simulink model "ENV_NEW"  (R2024b)
settings: Solver=FixedStepDiscrete  StartTime=0.0  StopTime=1  FixedStep=0.001  RelTol=1e-3  EnableMultiTasking=on
libraries: stm32blockslib x105, canmsglib x32, stm32f4xxblockslib x11, simulink x10
(part 2 of 5)

== system ENV_NEW/CAN RX ==
  Digital Port Read5 : stm32f4xxblockslib/Digital Port Read  PortName=GPIOB  PinNumber=PinNumber  ReadOperation=on  IOAsArray=off  SampleTime=-1  EnableSimPort=off  hoistedMaskSrc=ECSoC/ECSimCodegen/Digital Port Read
      settings: LibrarySourceBlock=stm32f2xxblockslib/Digital Port Read
  Enabled Subsystem : Subsystem  TreatAsAtomicUnit=on
  NOT5 : Logic  Operator=NOT  IconShape=distinctive  AllPortsSameDT=off  OutDataTypeStr=boolean
  CANMessage : Outport
  wires:
  NOT5/1 -> Enabled Subsystem/Enable
  Digital Port Read5/1 -> NOT5/1
  Enabled Subsystem/1(CANMessage) -> CANMessage/1

== system ENV_NEW/CAN RX1 ==
  Digital Port Read5 : stm32f4xxblockslib/Digital Port Read  PortName=GPIOC  PinNumber=PinNumber  ReadOperation=on  IOAsArray=off  SampleTime=-1  EnableSimPort=off  hoistedMaskSrc=ECSoC/ECSimCodegen/Digital Port Read
      settings: LibrarySourceBlock=stm32f2xxblockslib/Digital Port Read
  Enabled Subsystem : Subsystem  TreatAsAtomicUnit=on
  NOT5 : Logic  Operator=NOT  IconShape=distinctive  AllPortsSameDT=off  OutDataTypeStr=boolean
  CANMessage : Outport
  wires:
  NOT5/1 -> Enabled Subsystem/Enable
  Digital Port Read5/1 -> NOT5/1
  Enabled Subsystem/1(CANMessage) -> CANMessage/1

== system ENV_NEW/CAN RX2 ==
  Digital Port Read5 : stm32f4xxblockslib/Digital Port Read  PortName=GPIOA  PinNumber=PinNumber  ReadOperation=on  IOAsArray=off  SampleTime=-1  EnableSimPort=off  hoistedMaskSrc=ECSoC/ECSimCodegen/Digital Port Read
      settings: LibrarySourceBlock=stm32f2xxblockslib/Digital Port Read
  Enabled Subsystem : Subsystem  TreatAsAtomicUnit=on
  NOT5 : Logic  Operator=NOT  IconShape=distinctive  AllPortsSameDT=off  OutDataTypeStr=boolean
  CANMessage : Outport
  wires:
  NOT5/1 -> Enabled Subsystem/Enable
  Digital Port Read5/1 -> NOT5/1
  Enabled Subsystem/1(CANMessage) -> CANMessage/1

== system ENV_NEW/CAN RX3 ==
  Digital Port Read5 : stm32f4xxblockslib/Digital Port Read  PortName=GPIOC  PinNumber=PinNumber  ReadOperation=on  IOAsArray=off  SampleTime=-1  EnableSimPort=off  hoistedMaskSrc=ECSoC/ECSimCodegen/Digital Port Read
      settings: LibrarySourceBlock=stm32f2xxblockslib/Digital Port Read
  Enabled Subsystem : Subsystem  TreatAsAtomicUnit=on
  NOT5 : Logic  Operator=NOT  IconShape=distinctive  AllPortsSameDT=off  OutDataTypeStr=boolean
  CANMessage : Outport
  wires:
  NOT5/1 -> Enabled Subsystem/Enable
  Digital Port Read5/1 -> NOT5/1
  Enabled Subsystem/1(CANMessage) -> CANMessage/1

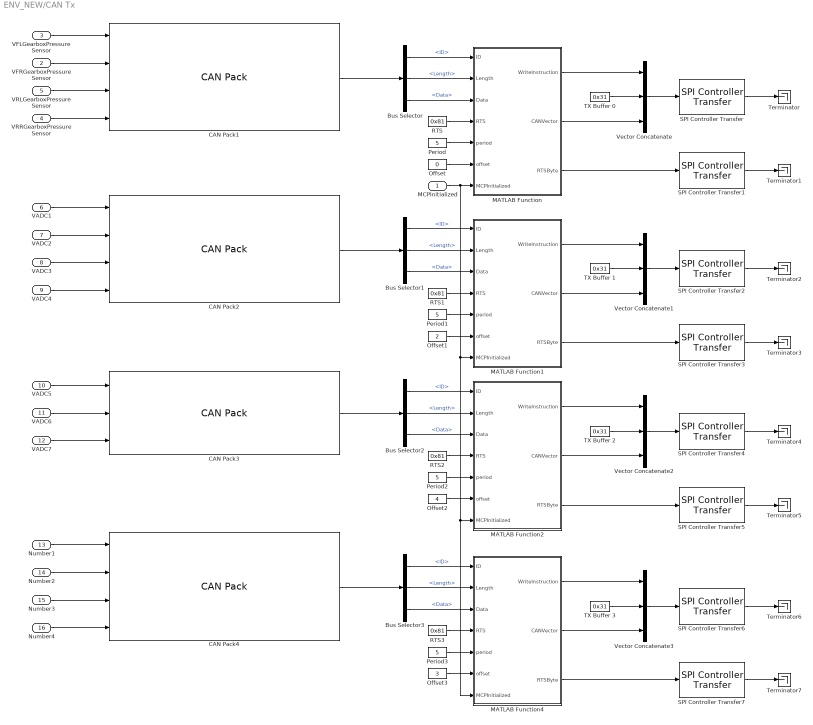
== system ENV_NEW/CAN Tx ==
  MCPInitialized : Inport
  VFRGearboxPressureSensor : Inport  Port=2
  VFLGearboxPressureSensor : Inport  Port=3
  VRRGearboxPressureSensor : Inport  Port=4
  VRLGearboxPressureSensor : Inport  Port=5
  VADC1 : Inport  Port=6
  VADC2 : Inport  Port=7
  VADC3 : Inport  Port=8
  VADC4 : Inport  Port=9
  VADC5 : Inport  Port=10
  VADC6 : Inport  Port=11
  VADC7 : Inport  Port=12
  Number1 : Inport  Port=13
  Number2 : Inport  Port=14
  Number3 : Inport  Port=15
  Number4 : Inport  Port=16
  Bus Selector{,1..3} (4 alike) : BusSelector  OutputSignals=ID,Length,Data
  CAN Pack1 : canmsglib/CAN Pack  CANdbFile=C:\Users\oxbro\Documents\STM32CustomProjects\PDUSTM32\ADCTest.dbc  MsgList=GearboxPressures  MsgName=GearboxPressures  MsgIDType=Standard (11-bit identifier)  MsgIdentifier=105  CANIDInput=off  MsgLength=8  Remote=off  ApplyMinMax=off  BusOutput=on  SignalInfo={'VFLGearboxPressureSensor','0','12','LE','unsigned','Standard','0','0.0012211','0','0','5.0004';'VFRGearboxPressureSensor','16','12','LE','unsigned','Standard','0','0.0012211','0','0','5.0004';'VRLGearboxPressureSensor','32','12','LE','unsigned','Standard','0','0.0012211','0','0','5.0004';'VRRGearboxPressureSensor','48','12','LE','unsigned','Standard','0','0.0012211','0','0','5.0004'}
      settings: LibrarySourceBlock=stmutilitieslib/CAN Pack  DataFormat=CANdb specified signals
  CAN Pack2 : canmsglib/CAN Pack  CANdbFile=C:\Users\oxbro\Documents\STM32CustomProjects\PDUSTM32\ADCTest.dbc  MsgList=ADCs1  MsgName=ADCs1  MsgIDType=Standard (11-bit identifier)  MsgIdentifier=5  CANIDInput=off  MsgLength=8  Remote=off  ApplyMinMax=off  BusOutput=on  SignalInfo={'VADC1','0','16','LE','unsigned','Standard','0','5.04e-05','0','0','3.303';'VADC2','16','16','LE','unsigned','Standard','0','5.04e-05','0','0','3.303';'VADC3','32','16','LE','unsigned','Standard','0','5.04e-05','0','0','3.303';'VADC4','48','16','LE','unsigned','Standard','0','5.04e-05','0','0','3.303'}
      settings: LibrarySourceBlock=stmutilitieslib/CAN Pack  DataFormat=CANdb specified signals
  CAN Pack3 : canmsglib/CAN Pack  CANdbFile=C:\Users\oxbro\Documents\STM32CustomProjects\PDUSTM32\ADCTest.dbc  MsgList=ADCs2  MsgName=ADCs2  MsgIDType=Standard (11-bit identifier)  MsgIdentifier=66  CANIDInput=off  MsgLength=6  Remote=off  ApplyMinMax=off  BusOutput=on  SignalInfo={'VADC5','0','16','LE','unsigned','Standard','0','5.04e-05','0','0','3.303';'VADC6','16','16','LE','unsigned','Standard','0','5.04e-05','0','0','3.303';'VLVSystem','32','16','LE','unsigned','Standard','0','0.00046327','0','0','30.3604'}
      settings: LibrarySourceBlock=stmutilitieslib/CAN Pack  DataFormat=CANdb specified signals
  CAN Pack4 : canmsglib/CAN Pack  CANdbFile=C:\Users\oxbro\Documents\STM32CustomProjects\PDUSTM32\ADCTest.dbc  MsgList=Numbers  MsgName=Numbers  MsgIDType=Standard (11-bit identifier)  MsgIdentifier=0  CANIDInput=off  MsgLength=8  Remote=off  ApplyMinMax=off  BusOutput=on  SignalInfo={'Number1','0','16','LE','signed','Standard','0','1','0','-32768','32767';'Number2','16','16','LE','signed','Standard','0','1','0','-32768','32767';'Number3','32','16','LE','signed','Standard','0','1','0','-32768','32767';'Number4','48','16','LE','signed','Standard','0','1','0','-32768','32767'}
      settings: LibrarySourceBlock=stmutilitieslib/CAN Pack  DataFormat=CANdb specified signals
  MATLAB Function : MATLAB Function  TreatAsAtomicUnit=on
  MATLAB Function1 : MATLAB Function  TreatAsAtomicUnit=on
  MATLAB Function2 : MATLAB Function  TreatAsAtomicUnit=on
  MATLAB Function4 : MATLAB Function  TreatAsAtomicUnit=on
  Offset : Constant  Value=0  OutDataTypeStr=uint16  SampleTime=-1
  Offset1 : Constant  Value=2  OutDataTypeStr=uint16  SampleTime=-1
  Offset2 : Constant  Value=4  OutDataTypeStr=uint16  SampleTime=-1
  Offset3 : Constant  Value=3  OutDataTypeStr=uint16  SampleTime=-1
  Period{,1..3} (4 alike) : Constant  Value=5  OutDataTypeStr=uint16  SampleTime=-1
  RTS{,1..3} (4 alike) : Constant  Value=0x81  OutDataTypeStr=uint8  SampleTime=-1
  SPI Controller Transfer{,2,4,6} (4 alike) : stm32blockslib/SPI Controller Transfer  Priority=1  SPIModuleSelect=SPI1  ClockPolarity=Low  ClockPhase=1 Edge  SPIModule=uint32(0)  Mode=Master  BusSpeed=uint32(1000000)  FirstBitToTransfer=Most significant bit (MSB)  ClockMode=0  BlockFunction=Transfer  EnableRegisterAddress=off  RegisterAddress=0  OutputDataType=uint8  OutputDataLength=1  OutputStatus=off  BlockingMode=off  Timeout=0.01  DataBits=8  UseCustomSSPin=Explicit GPIO calls  ActiveLowSSPin=Active low  Port_Select=GPIOA  Pin=1
      settings: LibrarySourceBlock=stm32h7xxblockslib/SPI Controller Transfer
  SPI Controller Transfer{1,3,5,7} (4 alike) : stm32blockslib/SPI Controller Transfer  Priority=2  SPIModuleSelect=SPI1  ClockPolarity=Low  ClockPhase=1 Edge  SPIModule=uint32(0)  Mode=Master  BusSpeed=uint32(1000000)  FirstBitToTransfer=Most significant bit (MSB)  ClockMode=0  BlockFunction=Transfer  EnableRegisterAddress=off  RegisterAddress=0  OutputDataType=uint8  OutputDataLength=1  OutputStatus=off  BlockingMode=off  Timeout=0.01  DataBits=8  UseCustomSSPin=Explicit GPIO calls  ActiveLowSSPin=Active low  Port_Select=GPIOA  Pin=1
      settings: LibrarySourceBlock=stm32h7xxblockslib/SPI Controller Transfer
  TX Buffer {0..3} (4 alike) : Constant  Value=0x31  OutDataTypeStr=uint8  SampleTime=-1
  Terminator{,1..7} (8 alike) : Terminator
  Vector Concatenate{,1..3} (4 alike) : Concatenate  NumInputs=3
  wires:
  SPI Controller Transfer/1 -> Terminator/1
  MATLAB Function/1(WriteInstruction) -> Vector Concatenate/1
  RTS/1 -> MATLAB Function/4(RTS)
  MATLAB Function/2(CANVector) -> Vector Concatenate/3
  SPI Controller Transfer1/1 -> Terminator1/1
  Bus Selector/1 -> MATLAB Function/1(ID)  "<ID>"
  Vector Concatenate/1 -> SPI Controller Transfer/1
  TX Buffer 0/1 -> Vector Concatenate/2
  MATLAB Function/3(RTSByte) -> SPI Controller Transfer1/1
  Bus Selector/2 -> MATLAB Function/2(Length)  "<Length>"
  Bus Selector/3 -> MATLAB Function/3(Data)  "<Data>"
  CAN Pack1/1 -> Bus Selector/1
  Period/1 -> MATLAB Function/5(period)
  Offset/1 -> MATLAB Function/6(offset)
  VRLGearboxPressureSensor/1 -> CAN Pack1/3
  VRRGearboxPressureSensor/1 -> CAN Pack1/4
  VFRGearboxPressureSensor/1 -> CAN Pack1/2
  VFLGearboxPressureSensor/1 -> CAN Pack1/1
  SPI Controller Transfer2/1 -> Terminator2/1
  SPI Controller Transfer3/1 -> Terminator3/1
  RTS1/1 -> MATLAB Function1/4(RTS)
  MATLAB Function1/2(CANVector) -> Vector Concatenate1/3
  Bus Selector1/3 -> MATLAB Function1/3(Data)  "<Data>"
  Period1/1 -> MATLAB Function1/5(period)
  Bus Selector1/2 -> MATLAB Function1/2(Length)  "<Length>"
  Offset1/1 -> MATLAB Function1/6(offset)
  CAN Pack2/1 -> Bus Selector1/1
  Bus Selector1/1 -> MATLAB Function1/1(ID)  "<ID>"
  MATLAB Function1/3(RTSByte) -> SPI Controller Transfer3/1
  Vector Concatenate1/1 -> SPI Controller Transfer2/1
  MATLAB Function1/1(WriteInstruction) -> Vector Concatenate1/1
  TX Buffer 1/1 -> Vector Concatenate1/2
  SPI Controller Transfer4/1 -> Terminator4/1
  SPI Controller Transfer5/1 -> Terminator5/1
  RTS2/1 -> MATLAB Function2/4(RTS)
  MATLAB Function2/2(CANVector) -> Vector Concatenate2/3
  Bus Selector2/3 -> MATLAB Function2/3(Data)  "<Data>"
  Period2/1 -> MATLAB Function2/5(period)
  Bus Selector2/2 -> MATLAB Function2/2(Length)  "<Length>"
  Offset2/1 -> MATLAB Function2/6(offset)
  CAN Pack3/1 -> Bus Selector2/1
  Bus Selector2/1 -> MATLAB Function2/1(ID)  "<ID>"
  MATLAB Function2/3(RTSByte) -> SPI Controller Transfer5/1
  Vector Concatenate2/1 -> SPI Controller Transfer4/1
  MATLAB Function2/1(WriteInstruction) -> Vector Concatenate2/1
  TX Buffer 2/1 -> Vector Concatenate2/2
  VADC1/1 -> CAN Pack2/1
  VADC2/1 -> CAN Pack2/2
  VADC3/1 -> CAN Pack2/3
  VADC4/1 -> CAN Pack2/4
  VADC5/1 -> CAN Pack3/1
  VADC6/1 -> CAN Pack3/2
  VADC7/1 -> CAN Pack3/3
  Period3/1 -> MATLAB Function4/5(period)
  Vector Concatenate3/1 -> SPI Controller Transfer6/1
  Offset3/1 -> MATLAB Function4/6(offset)
  Number1/1 -> CAN Pack4/1
  MATLAB Function4/3(RTSByte) -> SPI Controller Transfer7/1
  Number4/1 -> CAN Pack4/4
  MCPInitialized/1 -> MATLAB Function4/7(MCPInitialized), MATLAB Function2/7(MCPInitialized), MATLAB Function1/7(MCPInitialized), MATLAB Function/7(MCPInitialized)
  MATLAB Function4/2(CANVector) -> Vector Concatenate3/3
  Number3/1 -> CAN Pack4/3
  Bus Selector3/3 -> MATLAB Function4/3(Data)  "<Data>"
  Number2/1 -> CAN Pack4/2
  CAN Pack4/1 -> Bus Selector3/1
  Bus Selector3/1 -> MATLAB Function4/1(ID)  "<ID>"
  MATLAB Function4/1(WriteInstruction) -> Vector Concatenate3/1
  TX Buffer 3/1 -> Vector Concatenate3/2
  SPI Controller Transfer6/1 -> Terminator6/1
  SPI Controller Transfer7/1 -> Terminator7/1
  Bus Selector3/2 -> MATLAB Function4/2(Length)  "<Length>"
  RTS3/1 -> MATLAB Function4/4(RTS)

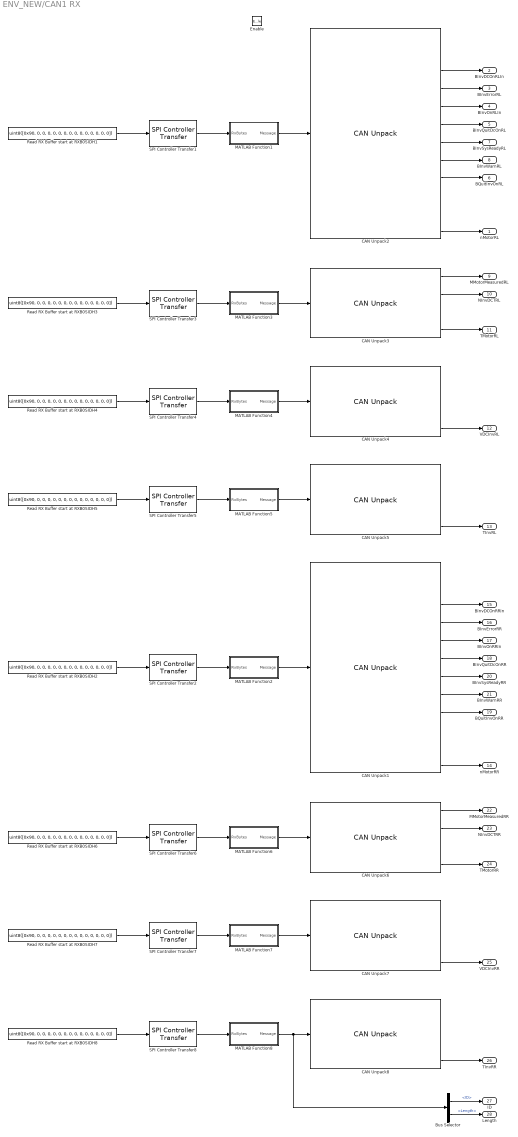
== system ENV_NEW/CAN1 RX ==
  Enable : EnablePort
  Bus Selector : BusSelector  OutputSignals=ID,Length
  CAN Unpack1 : canmsglib/CAN Unpack  CANdbFile=C:\Users\Will\Desktop\OBR\Embedded\VCUSTM32\Controls\CAN\Inverters\26.06.18_CAN1.dbc  MsgList=INV3_Send_1  MsgName=INV3_Send_1  MsgIDType=Standard (11-bit identifier)  MsgIdentifier=644  MsgLength=8  SignalInfo={'AMK_bDerating','47','1','LE','unsigned','Standard','0','1','0','0','1';'AMK_bReserve','32','8','LE','signed','Standard','0','1','0','-128','127';'BInvDCOnRRIn','44','1','LE','unsigned','Standard','0','1','0','0','1';'BInvErrorRR','41','1','LE','unsigned','Standard','0','1','0','0','1';'BInvOnRRIn','46','1','LE','unsigned','Standard','0','1','0','0','1';'BInvQuitDcOnRR','43','1','LE','unsigned','Standard','0','1','0','0','1';'BInvSysReadyRR','40','1','LE','unsigned','Standard','0','1','0','0','1';'BInvWarnRR','42','1','LE','unsigned','Standard','0','1','0','0','1';'BQuitInvOnRR','45','1','LE','unsigned','Standard','0','1','0','0','1';'Checksum','16','16','LE','unsigned','Standard','0','1','0','0','65535';'Message_Counter','0','16','LE','unsigned','Standard','0','1','0','0','65535';'nMotorRR','48','16','LE','signed','Standard','0','1','0','-32768','32767'}  IDPort=off  TimestampPort=off  ErrorPort=off  RemotePort=off  LengthPort=off  StatusPort=off  ApplyMinMax=off
      settings: LibrarySourceBlock=stmutilitieslib/CAN Unpack  DataFormat=CANdb specified signals
  CAN Unpack2 : canmsglib/CAN Unpack  CANdbFile=C:\Users\Will\Desktop\OBR\Embedded\VCUSTM32\Controls\CAN\Inverters\26.06.18_CAN1.dbc  MsgList=INV1_Send_1  MsgName=INV1_Send_1  MsgIDType=Standard (11-bit identifier)  MsgIdentifier=643  MsgLength=8  SignalInfo={'AMK_bDerating','47','1','LE','unsigned','Standard','0','1','0','0','1';'AMK_bReserve','32','8','LE','signed','Standard','0','1','0','-128','127';'BInvDCOnRLIn','44','1','LE','unsigned','Standard','0','1','0','0','1';'BInvErrorRL','41','1','LE','unsigned','Standard','0','1','0','0','1';'BInvOnRLIn','46','1','LE','unsigned','Standard','0','1','0','0','1';'BInvQuitDcOnRL','43','1','LE','unsigned','Standard','0','1','0','0','1';'BInvSysReadyRL','40','1','LE','unsigned','Standard','0','1','0','0','1';'BInvWarnRL','42','1','LE','unsigned','Standard','0','1','0','0','1';'BQuitInvOnRL','45','1','LE','unsigned','Standard','0','1','0','0','1';'Checksum','16','16','LE','unsigned','Standard','0','1','0','0','65535';'Message_Counter','0','16','LE','unsigned','Standard','0','1','0','0','65535';'nMotorRL','48','16','LE','signed','Standard','0','1','0','-32768','32767'}  IDPort=off  TimestampPort=off  ErrorPort=off  RemotePort=off  LengthPort=off  StatusPort=off  ApplyMinMax=off
      settings: LibrarySourceBlock=stmutilitieslib/CAN Unpack  DataFormat=CANdb specified signals
  CAN Unpack3 : canmsglib/CAN Unpack  CANdbFile=C:\Users\Will\Desktop\OBR\Embedded\VCUSTM32\Controls\CAN\Inverters\26.06.18_CAN1.dbc  MsgList=INV1_Send_2  MsgName=INV1_Send_2  MsgIDType=Standard (11-bit identifier)  MsgIdentifier=645  MsgLength=8  SignalInfo={'MMotorMeasuredRL','16','16','LE','signed','Standard','0','1','0','-32768','32767';'NInvDTCRL','32','16','LE','signed','Standard','0','1','0','-32768','32767';'NInvErrorInfoRL1','48','16','LE','signed','Standard','0','1','0','-32768','32767';'TMotorRL','0','16','LE','signed','Standard','0','0.1','0','-3276.8','3276.7'}  IDPort=off  TimestampPort=off  ErrorPort=off  RemotePort=off  LengthPort=off  StatusPort=off  ApplyMinMax=off
      settings: LibrarySourceBlock=stmutilitieslib/CAN Unpack  DataFormat=CANdb specified signals
  CAN Unpack4 : canmsglib/CAN Unpack  CANdbFile=C:\Users\Will\Desktop\OBR\Embedded\VCUSTM32\Controls\CAN\Inverters\26.06.18_CAN1.dbc  MsgList=INV1_Send_3  MsgName=INV1_Send_3  MsgIDType=Standard (11-bit identifier)  MsgIdentifier=647  MsgLength=8  SignalInfo={'NInvErrorInfoRL2','0','16','LE','signed','Standard','0','1','0','-32768','32767';'NInvErrorInfoRL3','16','16','LE','signed','Standard','0','1','0','-32768','32767';'Raw_Torque_Current','32','16','LE','signed','Standard','0','1','0','-32768','32767';'VDCInvRL','48','16','LE','signed','Standard','0','1','0','-32768','32767'}  IDPort=off  TimestampPort=off  ErrorPort=off  RemotePort=off  LengthPort=off  StatusPort=off  ApplyMinMax=off
      settings: LibrarySourceBlock=stmutilitieslib/CAN Unpack  DataFormat=CANdb specified signals
  CAN Unpack5 : canmsglib/CAN Unpack  CANdbFile=C:\Users\Will\Desktop\OBR\Embedded\VCUSTM32\Controls\CAN\Inverters\26.06.18_CAN1.dbc  MsgList=INV1_Send_4  MsgName=INV1_Send_4  MsgIDType=Standard (11-bit identifier)  MsgIdentifier=649  MsgLength=8  SignalInfo={'Converter_Peak_Current','32','16','LE','signed','Standard','0','1','0','-32768','32767';'Motor_Nomial_Current_IN','48','16','LE','signed','Standard','0','1','0','-32768','32767';'Motor_Peak_Current','16','16','LE','signed','Standard','0','1','0','-32768','32767';'TInvRL','0','16','LE','signed','Standard','0','0.1','0','-3276.8','3276.7'}  IDPort=off  TimestampPort=off  ErrorPort=off  RemotePort=off  LengthPort=off  StatusPort=off  ApplyMinMax=off
      settings: LibrarySourceBlock=stmutilitieslib/CAN Unpack  DataFormat=CANdb specified signals
  CAN Unpack6 : canmsglib/CAN Unpack  CANdbFile=C:\Users\Will\Desktop\OBR\Embedded\VCUSTM32\Controls\CAN\Inverters\26.06.18_CAN1.dbc  MsgList=INV3_Send_2  MsgName=INV3_Send_2  MsgIDType=Standard (11-bit identifier)  MsgIdentifier=646  MsgLength=8  SignalInfo={'MMotorMeasuredRR','16','16','LE','signed','Standard','0','1','0','-32768','32767';'NInvDTCRR','32','16','LE','signed','Standard','0','1','0','-32768','32767';'NInvErrorInfoRR1','48','16','LE','signed','Standard','0','1','0','-32768','32767';'TMotorRR','0','16','LE','signed','Standard','0','0.1','0','-3276.8','3276.7'}  IDPort=off  TimestampPort=off  ErrorPort=off  RemotePort=off  LengthPort=off  StatusPort=off  ApplyMinMax=off
      settings: LibrarySourceBlock=stmutilitieslib/CAN Unpack  DataFormat=CANdb specified signals
  CAN Unpack7 : canmsglib/CAN Unpack  CANdbFile=C:\Users\Will\Desktop\OBR\Embedded\VCUSTM32\Controls\CAN\Inverters\26.06.18_CAN1.dbc  MsgList=INV3_Send_3  MsgName=INV3_Send_3  MsgIDType=Standard (11-bit identifier)  MsgIdentifier=648  MsgLength=8  SignalInfo={'NInvErrorInfoRR2','0','16','LE','signed','Standard','0','1','0','-32768','32767';'NInvErrorInfoRR3','16','16','LE','signed','Standard','0','1','0','-32768','32767';'Raw_Torque_Current','32','16','LE','signed','Standard','0','1','0','-32768','32767';'VDCInvRR','48','16','LE','signed','Standard','0','1','0','-32768','32767'}  IDPort=off  TimestampPort=off  ErrorPort=off  RemotePort=off  LengthPort=off  StatusPort=off  ApplyMinMax=off
      settings: LibrarySourceBlock=stmutilitieslib/CAN Unpack  DataFormat=CANdb specified signals
  CAN Unpack8 : canmsglib/CAN Unpack  CANdbFile=C:\Users\Will\Desktop\OBR\Embedded\VCUSTM32\Controls\CAN\Inverters\26.06.18_CAN1.dbc  MsgList=INV3_Send_4  MsgName=INV3_Send_4  MsgIDType=Standard (11-bit identifier)  MsgIdentifier=656  MsgLength=8  SignalInfo={'Converter_Peak_Current','32','16','LE','signed','Standard','0','1','0','-32768','32767';'Motor_Nomial_Current_IN','48','16','LE','signed','Standard','0','1','0','-32768','32767';'Motor_Peak_Current','16','16','LE','signed','Standard','0','1','0','-32768','32767';'TInvRR','0','16','LE','signed','Standard','0','0.1','0','-3276.8','3276.7'}  IDPort=off  TimestampPort=off  ErrorPort=off  RemotePort=off  LengthPort=off  StatusPort=off  ApplyMinMax=off
      settings: LibrarySourceBlock=stmutilitieslib/CAN Unpack  DataFormat=CANdb specified signals
  MATLAB Function1 : MATLAB Function  TreatAsAtomicUnit=on
  MATLAB Function2 : MATLAB Function  TreatAsAtomicUnit=on
  MATLAB Function3 : MATLAB Function  TreatAsAtomicUnit=on
  MATLAB Function4 : MATLAB Function  TreatAsAtomicUnit=on
  MATLAB Function5 : MATLAB Function  TreatAsAtomicUnit=on
  MATLAB Function6 : MATLAB Function  TreatAsAtomicUnit=on
  MATLAB Function7 : MATLAB Function  TreatAsAtomicUnit=on
  MATLAB Function8 : MATLAB Function  TreatAsAtomicUnit=on
  Read RX Buffer start at RXB0SIDH{1..8} (8 alike) : Constant  Value=uint8([0x90, 0, 0, 0, 0, 0, 0, 0, 0, 0, 0, 0, 0, 0, 0])
  SPI Controller Transfer{1..8} (8 alike) : stm32blockslib/SPI Controller Transfer  Priority=1  SPIModuleSelect=SPI1  ClockPolarity=Low  ClockPhase=1 Edge  SPIModule=uint32(0)  Mode=Master  BusSpeed=uint32(1000000)  FirstBitToTransfer=Most significant bit (MSB)  ClockMode=0  BlockFunction=Transfer  EnableRegisterAddress=off  RegisterAddress=0  OutputDataType=uint8  OutputDataLength=1  OutputStatus=off  BlockingMode=on  Timeout=0.01  DataBits=8  UseCustomSSPin=Explicit GPIO calls  ActiveLowSSPin=Active low  Port_Select=GPIOB  Pin=1
      settings: LibrarySourceBlock=stm32h7xxblockslib/SPI Controller Transfer
  nMotorRL : Outport  OutDataTypeStr=double
  BInvDCOnRLIn : Outport  Port=2  OutDataTypeStr=boolean
  BInvErrorRL : Outport  Port=3  OutDataTypeStr=boolean
  BInvOnRLIn : Outport  Port=4  OutDataTypeStr=boolean
  BInvQuitDcOnRL : Outport  Port=5  OutDataTypeStr=boolean
  BQuitInvOnRL : Outport  Port=6  OutDataTypeStr=boolean
  BInvSysReadyRL : Outport  Port=7  OutDataTypeStr=boolean
  BInvWarnRL : Outport  Port=8  OutDataTypeStr=boolean
  MMotorMeasuredRL : Outport  Port=9  OutDataTypeStr=double
  NInvDCTRL : Outport  Port=10  OutDataTypeStr=double
  TMotorRL : Outport  Port=11  OutDataTypeStr=double
  VDCInvRL : Outport  Port=12  OutDataTypeStr=double
  TInvRL : Outport  Port=13  OutDataTypeStr=double
  nMotorRR : Outport  Port=14  OutDataTypeStr=double
  BInvDCOnRRIn : Outport  Port=15  OutDataTypeStr=boolean
  BInvErrorRR : Outport  Port=16  OutDataTypeStr=boolean
  BInvOnRRIn : Outport  Port=17  OutDataTypeStr=boolean
  BInvQuitDcOnRR : Outport  Port=18  OutDataTypeStr=boolean
  BQuitInvOnRR : Outport  Port=19  OutDataTypeStr=boolean
  BInvSysReadyRR : Outport  Port=20  OutDataTypeStr=boolean
  BInvWarnRR : Outport  Port=21  OutDataTypeStr=boolean
  MMotorMeasuredRR : Outport  Port=22  OutDataTypeStr=double
  NInvDCTRR : Outport  Port=23  OutDataTypeStr=double
  TMotorRR : Outport  Port=24  OutDataTypeStr=double
  VDCInvRR : Outport  Port=25  OutDataTypeStr=double
  TInvRR : Outport  Port=26  OutDataTypeStr=double
  ID : Outport  Port=27
  Length : Outport  Port=28
  wires:
  Read RX Buffer start at RXB0SIDH1/1 -> SPI Controller Transfer1/1
  SPI Controller Transfer1/1 -> MATLAB Function1/1(RxBytes)
  MATLAB Function1/1(Message) -> CAN Unpack2/1
  CAN Unpack2/3 -> BInvDCOnRLIn/1
  CAN Unpack2/4 -> BInvErrorRL/1
  CAN Unpack2/5 -> BInvOnRLIn/1
  CAN Unpack2/6 -> BInvQuitDcOnRL/1
  CAN Unpack2/9 -> BQuitInvOnRL/1
  CAN Unpack2/8 -> BInvWarnRL/1
  CAN Unpack2/7 -> BInvSysReadyRL/1
  CAN Unpack2/12 -> nMotorRL/1
  CAN Unpack3/4 -> TMotorRL/1
  MATLAB Function3/1(Message) -> CAN Unpack3/1
  SPI Controller Transfer3/1 -> MATLAB Function3/1(RxBytes)
  Read RX Buffer start at RXB0SIDH3/1 -> SPI Controller Transfer3/1
  CAN Unpack3/1 -> MMotorMeasuredRL/1
  CAN Unpack3/2 -> NInvDCTRL/1
  CAN Unpack4/4 -> VDCInvRL/1
  SPI Controller Transfer4/1 -> MATLAB Function4/1(RxBytes)
  MATLAB Function4/1(Message) -> CAN Unpack4/1
  Read RX Buffer start at RXB0SIDH4/1 -> SPI Controller Transfer4/1
  SPI Controller Transfer5/1 -> MATLAB Function5/1(RxBytes)
  CAN Unpack5/4 -> TInvRL/1
  Read RX Buffer start at RXB0SIDH5/1 -> SPI Controller Transfer5/1
  MATLAB Function5/1(Message) -> CAN Unpack5/1
  MATLAB Function8/1(Message) -> CAN Unpack8/1, Bus Selector/1
  Bus Selector/2 -> Length/1  "<Length>"
  Bus Selector/1 -> ID/1  "<ID>"
  CAN Unpack1/6 -> BInvQuitDcOnRR/1
  CAN Unpack1/3 -> BInvDCOnRRIn/1
  CAN Unpack6/4 -> TMotorRR/1
  CAN Unpack1/5 -> BInvOnRRIn/1
  SPI Controller Transfer2/1 -> MATLAB Function2/1(RxBytes)
  MATLAB Function2/1(Message) -> CAN Unpack1/1
  SPI Controller Transfer8/1 -> MATLAB Function8/1(RxBytes)
  CAN Unpack1/8 -> BInvWarnRR/1
  CAN Unpack6/1 -> MMotorMeasuredRR/1
  CAN Unpack1/12 -> nMotorRR/1
  CAN Unpack1/4 -> BInvErrorRR/1
  CAN Unpack1/7 -> BInvSysReadyRR/1
  CAN Unpack1/9 -> BQuitInvOnRR/1
  Read RX Buffer start at RXB0SIDH2/1 -> SPI Controller Transfer2/1
  SPI Controller Transfer7/1 -> MATLAB Function7/1(RxBytes)
  Read RX Buffer start at RXB0SIDH8/1 -> SPI Controller Transfer8/1
  MATLAB Function6/1(Message) -> CAN Unpack6/1
  Read RX Buffer start at RXB0SIDH7/1 -> SPI Controller Transfer7/1
  CAN Unpack6/2 -> NInvDCTRR/1
  SPI Controller Transfer6/1 -> MATLAB Function6/1(RxBytes)
  MATLAB Function7/1(Message) -> CAN Unpack7/1
  Read RX Buffer start at RXB0SIDH6/1 -> SPI Controller Transfer6/1
  CAN Unpack7/4 -> VDCInvRR/1
  CAN Unpack8/4 -> TInvRR/1

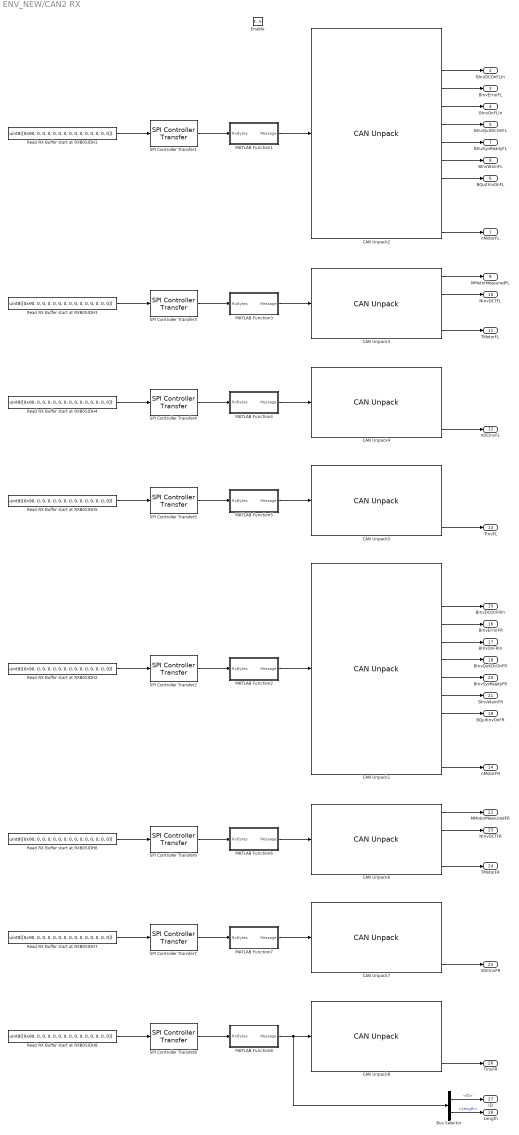
== system ENV_NEW/CAN2 RX ==
  Enable : EnablePort
  Bus Selector : BusSelector  OutputSignals=ID,Length
  CAN Unpack1 : canmsglib/CAN Unpack  CANdbFile=C:\Users\Will\Desktop\OBR\Embedded\VCUSTM32\Controls\CAN\Inverters\26.06.18_CAN2.dbc  MsgList=INV4_Send_1  MsgName=INV4_Send_1  MsgIDType=Standard (11-bit identifier)  MsgIdentifier=658  MsgLength=8  SignalInfo={'AMK_bDerating','47','1','LE','unsigned','Standard','0','1','0','0','1';'AMK_bReserve','32','8','LE','signed','Standard','0','1','0','-128','127';'BInvDCOnFRIn','44','1','LE','unsigned','Standard','0','1','0','0','1';'BInvErrorFR','41','1','LE','unsigned','Standard','0','1','0','0','1';'BInvOnFRIn','46','1','LE','unsigned','Standard','0','1','0','0','1';'BInvQuitDcOnFR','43','1','LE','unsigned','Standard','0','1','0','0','1';'BInvSysReadyFR','40','1','LE','unsigned','Standard','0','1','0','0','1';'BInvWarnFR','42','1','LE','unsigned','Standard','0','1','0','0','1';'BQuitInvOnFR','45','1','LE','unsigned','Standard','0','1','0','0','1';'Checksum','16','16','LE','unsigned','Standard','0','1','0','0','65535';'Message_Counter','0','16','LE','unsigned','Standard','0','1','0','0','65535';'nMotorFR','48','16','LE','signed','Standard','0','1','0','-32768','32767'}  IDPort=off  TimestampPort=off  ErrorPort=off  RemotePort=off  LengthPort=off  StatusPort=off  ApplyMinMax=off
      settings: LibrarySourceBlock=stmutilitieslib/CAN Unpack  DataFormat=CANdb specified signals
  CAN Unpack2 : canmsglib/CAN Unpack  CANdbFile=C:\Users\Will\Desktop\OBR\Embedded\VCUSTM32\Controls\CAN\Inverters\26.06.18_CAN2.dbc  MsgList=INV2_Send_1  MsgName=INV2_Send_1  MsgIDType=Standard (11-bit identifier)  MsgIdentifier=657  MsgLength=8  SignalInfo={'AMK_bDerating','47','1','LE','unsigned','Standard','0','1','0','0','1';'AMK_bReserve','32','8','LE','signed','Standard','0','1','0','-128','127';'BInvDCOnFLIn','44','1','LE','unsigned','Standard','0','1','0','0','1';'BInvErrorFL','41','1','LE','unsigned','Standard','0','1','0','0','1';'BInvOnFLIn','46','1','LE','unsigned','Standard','0','1','0','0','1';'BInvQuitDcOnFL','43','1','LE','unsigned','Standard','0','1','0','0','1';'BInvSysReadyFL','40','1','LE','unsigned','Standard','0','1','0','0','1';'BInvWarnFL','42','1','LE','unsigned','Standard','0','1','0','0','1';'BQuitInvOnFL','45','1','LE','unsigned','Standard','0','1','0','0','1';'Checksum','16','16','LE','unsigned','Standard','0','1','0','0','65535';'Message_Counter','0','16','LE','unsigned','Standard','0','1','0','0','65535';'nMotorFL','48','16','LE','signed','Standard','0','1','0','-32768','32767'}  IDPort=off  TimestampPort=off  ErrorPort=off  RemotePort=off  LengthPort=off  StatusPort=off  ApplyMinMax=off
      settings: LibrarySourceBlock=stmutilitieslib/CAN Unpack  DataFormat=CANdb specified signals
  CAN Unpack3 : canmsglib/CAN Unpack  CANdbFile=C:\Users\Will\Desktop\OBR\Embedded\VCUSTM32\Controls\CAN\Inverters\26.06.18_CAN2.dbc  MsgList=INV2_Send_2  MsgName=INV2_Send_2  MsgIDType=Standard (11-bit identifier)  MsgIdentifier=659  MsgLength=8  SignalInfo={'MMotorMeasuredFL','16','16','LE','signed','Standard','0','1','0','-32768','32767';'NInvDTCFL','32','16','LE','signed','Standard','0','1','0','-32768','32767';'NInvErrorInfoFL1','48','16','LE','signed','Standard','0','1','0','-32768','32767';'TMotorFL','0','16','LE','signed','Standard','0','0.1','0','-3276.8','3276.7'}  IDPort=off  TimestampPort=off  ErrorPort=off  RemotePort=off  LengthPort=off  StatusPort=off  ApplyMinMax=off
      settings: LibrarySourceBlock=stmutilitieslib/CAN Unpack  DataFormat=CANdb specified signals
  CAN Unpack4 : canmsglib/CAN Unpack  CANdbFile=C:\Users\Will\Desktop\OBR\Embedded\VCUSTM32\Controls\CAN\Inverters\26.06.18_CAN2.dbc  MsgList=INV2_Send_3  MsgName=INV2_Send_3  MsgIDType=Standard (11-bit identifier)  MsgIdentifier=661  MsgLength=8  SignalInfo={'NInvErrorInfoFL2','0','16','LE','signed','Standard','0','1','0','-32768','32767';'NInvErrorInfoFL3','16','16','LE','signed','Standard','0','1','0','-32768','32767';'Raw_Torque_Current','32','16','LE','signed','Standard','0','1','0','-32768','32767';'VDCInvFL','48','16','LE','signed','Standard','0','1','0','-32768','32767'}  IDPort=off  TimestampPort=off  ErrorPort=off  RemotePort=off  LengthPort=off  StatusPort=off  ApplyMinMax=off
      settings: LibrarySourceBlock=stmutilitieslib/CAN Unpack  DataFormat=CANdb specified signals
  CAN Unpack5 : canmsglib/CAN Unpack  CANdbFile=C:\Users\Will\Desktop\OBR\Embedded\VCUSTM32\Controls\CAN\Inverters\26.06.18_CAN2.dbc  MsgList=INV2_Send_4  MsgName=INV2_Send_4  MsgIDType=Standard (11-bit identifier)  MsgIdentifier=663  MsgLength=8  SignalInfo={'Converter_Peak_Current','32','16','LE','signed','Standard','0','1','0','-32768','32767';'Motor_Nomial_Current_IN','48','16','LE','signed','Standard','0','1','0','-32768','32767';'Motor_Peak_Current','16','16','LE','signed','Standard','0','1','0','-32768','32767';'TInvFL','0','16','LE','signed','Standard','0','0.1','0','-3276.8','3276.7'}  IDPort=off  TimestampPort=off  ErrorPort=off  RemotePort=off  LengthPort=off  StatusPort=off  ApplyMinMax=off
      settings: LibrarySourceBlock=stmutilitieslib/CAN Unpack  DataFormat=CANdb specified signals
  CAN Unpack6 : canmsglib/CAN Unpack  CANdbFile=C:\Users\Will\Desktop\OBR\Embedded\VCUSTM32\Controls\CAN\Inverters\26.06.18_CAN2.dbc  MsgList=INV4_Send_2  MsgName=INV4_Send_2  MsgIDType=Standard (11-bit identifier)  MsgIdentifier=660  MsgLength=8  SignalInfo={'MMotorMeasuredFR','16','16','LE','signed','Standard','0','1','0','-32768','32767';'NInvDTCFR','32','16','LE','signed','Standard','0','1','0','-32768','32767';'NInvErrorInfoFR1','48','16','LE','signed','Standard','0','1','0','-32768','32767';'TMotorFR','0','16','LE','signed','Standard','0','0.1','0','-3276.8','3276.7'}  IDPort=off  TimestampPort=off  ErrorPort=off  RemotePort=off  LengthPort=off  StatusPort=off  ApplyMinMax=off
      settings: LibrarySourceBlock=stmutilitieslib/CAN Unpack  DataFormat=CANdb specified signals
  CAN Unpack7 : canmsglib/CAN Unpack  CANdbFile=C:\Users\Will\Desktop\OBR\Embedded\VCUSTM32\Controls\CAN\Inverters\26.06.18_CAN2.dbc  MsgList=INV4_Send_3  MsgName=INV4_Send_3  MsgIDType=Standard (11-bit identifier)  MsgIdentifier=662  MsgLength=8  SignalInfo={'NInvErrorInfoFR2','0','16','LE','signed','Standard','0','1','0','-32768','32767';'NInvErrorInfoFR3','16','16','LE','signed','Standard','0','1','0','-32768','32767';'Raw_Torque_Current','32','16','LE','signed','Standard','0','1','0','-32768','32767';'VDCInvFR','48','16','LE','signed','Standard','0','1','0','-32768','32767'}  IDPort=off  TimestampPort=off  ErrorPort=off  RemotePort=off  LengthPort=off  StatusPort=off  ApplyMinMax=off
      settings: LibrarySourceBlock=stmutilitieslib/CAN Unpack  DataFormat=CANdb specified signals
  CAN Unpack8 : canmsglib/CAN Unpack  CANdbFile=C:\Users\Will\Desktop\OBR\Embedded\VCUSTM32\Controls\CAN\Inverters\26.06.18_CAN2.dbc  MsgList=INV4_Send_4  MsgName=INV4_Send_4  MsgIDType=Standard (11-bit identifier)  MsgIdentifier=664  MsgLength=8  SignalInfo={'Converter_Peak_Current','32','16','LE','signed','Standard','0','1','0','-32768','32767';'Motor_Nomial_Current_IN','48','16','LE','signed','Standard','0','1','0','-32768','32767';'Motor_Peak_Current','16','16','LE','signed','Standard','0','1','0','-32768','32767';'TInvFR','0','16','LE','signed','Standard','0','0.1','0','-3276.8','3276.7'}  IDPort=off  TimestampPort=off  ErrorPort=off  RemotePort=off  LengthPort=off  StatusPort=off  ApplyMinMax=off
      settings: LibrarySourceBlock=stmutilitieslib/CAN Unpack  DataFormat=CANdb specified signals
  MATLAB Function1 : MATLAB Function  TreatAsAtomicUnit=on
  MATLAB Function2 : MATLAB Function  TreatAsAtomicUnit=on
  MATLAB Function3 : MATLAB Function  TreatAsAtomicUnit=on
  MATLAB Function4 : MATLAB Function  TreatAsAtomicUnit=on
  MATLAB Function5 : MATLAB Function  TreatAsAtomicUnit=on
  MATLAB Function6 : MATLAB Function  TreatAsAtomicUnit=on
  MATLAB Function7 : MATLAB Function  TreatAsAtomicUnit=on
  MATLAB Function8 : MATLAB Function  TreatAsAtomicUnit=on
  Read RX Buffer start at RXB0SIDH{1..8} (8 alike) : Constant  Value=uint8([0x90, 0, 0, 0, 0, 0, 0, 0, 0, 0, 0, 0, 0, 0, 0])
  SPI Controller Transfer{1..8} (8 alike) : stm32blockslib/SPI Controller Transfer  Priority=1  SPIModuleSelect=SPI1  ClockPolarity=Low  ClockPhase=1 Edge  SPIModule=uint32(0)  Mode=Master  BusSpeed=uint32(1000000)  FirstBitToTransfer=Most significant bit (MSB)  ClockMode=0  BlockFunction=Transfer  EnableRegisterAddress=off  RegisterAddress=0  OutputDataType=uint8  OutputDataLength=1  OutputStatus=off  BlockingMode=on  Timeout=0.01  DataBits=8  UseCustomSSPin=Explicit GPIO calls  ActiveLowSSPin=Active low  Port_Select=GPIOC  Pin=10
      settings: LibrarySourceBlock=stm32h7xxblockslib/SPI Controller Transfer
  nMotorFL : Outport  OutDataTypeStr=double
  BInvDCOnFLIn : Outport  Port=2  OutDataTypeStr=boolean
  BInvErrorFL : Outport  Port=3  OutDataTypeStr=boolean
  BInvOnFLIn : Outport  Port=4  OutDataTypeStr=boolean
  BInvQuitDcOnFL : Outport  Port=5  OutDataTypeStr=boolean
  BQuitInvOnFL : Outport  Port=6  OutDataTypeStr=boolean
  BInvSysReadyFL : Outport  Port=7  OutDataTypeStr=boolean
  BInvWarnFL : Outport  Port=8  OutDataTypeStr=boolean
  MMotorMeasuredFL : Outport  Port=9  OutDataTypeStr=double
  NInvDCTFL : Outport  Port=10  OutDataTypeStr=double
  TMotorFL : Outport  Port=11  OutDataTypeStr=double
  VDCInvFL : Outport  Port=12  OutDataTypeStr=double
  TInvFL : Outport  Port=13  OutDataTypeStr=double
  nMotorFR : Outport  Port=14  OutDataTypeStr=double
  BInvDCOnFRIn : Outport  Port=15  OutDataTypeStr=boolean
  BInvErrorFR : Outport  Port=16  OutDataTypeStr=boolean
  BInvOnFRIn : Outport  Port=17  OutDataTypeStr=boolean
  BInvQuitDcOnFR : Outport  Port=18  OutDataTypeStr=boolean
  BQuitInvOnFR : Outport  Port=19  OutDataTypeStr=boolean
  BInvSysReadyFR : Outport  Port=20  OutDataTypeStr=boolean
  BInvWarnFR : Outport  Port=21  OutDataTypeStr=boolean
  MMotorMeasuredFR : Outport  Port=22  OutDataTypeStr=double
  NInvDCTFR : Outport  Port=23  OutDataTypeStr=double
  TMotorFR : Outport  Port=24  OutDataTypeStr=double
  VDCInvFR : Outport  Port=25  OutDataTypeStr=double
  TInvFR : Outport  Port=26  OutDataTypeStr=double
  ID : Outport  Port=27
  Length : Outport  Port=28
  wires:
  Read RX Buffer start at RXB0SIDH1/1 -> SPI Controller Transfer1/1
  SPI Controller Transfer1/1 -> MATLAB Function1/1(RxBytes)
  MATLAB Function1/1(Message) -> CAN Unpack2/1
  CAN Unpack2/3 -> BInvDCOnFLIn/1
  CAN Unpack2/4 -> BInvErrorFL/1
  CAN Unpack2/5 -> BInvOnFLIn/1
  CAN Unpack2/6 -> BInvQuitDcOnFL/1
  CAN Unpack2/9 -> BQuitInvOnFL/1
  CAN Unpack2/8 -> BInvWarnFL/1
  CAN Unpack2/7 -> BInvSysReadyFL/1
  CAN Unpack2/12 -> nMotorFL/1
  CAN Unpack3/4 -> TMotorFL/1
  MATLAB Function3/1(Message) -> CAN Unpack3/1
  SPI Controller Transfer3/1 -> MATLAB Function3/1(RxBytes)
  Read RX Buffer start at RXB0SIDH3/1 -> SPI Controller Transfer3/1
  CAN Unpack3/1 -> MMotorMeasuredFL/1
  CAN Unpack3/2 -> NInvDCTFL/1
  CAN Unpack4/4 -> VDCInvFL/1
  SPI Controller Transfer4/1 -> MATLAB Function4/1(RxBytes)
  MATLAB Function4/1(Message) -> CAN Unpack4/1
  Read RX Buffer start at RXB0SIDH4/1 -> SPI Controller Transfer4/1
  SPI Controller Transfer5/1 -> MATLAB Function5/1(RxBytes)
  CAN Unpack5/4 -> TInvFL/1
  Read RX Buffer start at RXB0SIDH5/1 -> SPI Controller Transfer5/1
  MATLAB Function5/1(Message) -> CAN Unpack5/1
  MATLAB Function8/1(Message) -> Bus Selector/1, CAN Unpack8/1
  Bus Selector/2 -> Length/1  "<Length>"
  Bus Selector/1 -> ID/1  "<ID>"
  CAN Unpack1/6 -> BInvQuitDcOnFR/1
  CAN Unpack1/3 -> BInvDCOnFRIn/1
  CAN Unpack6/4 -> TMotorFR/1
  CAN Unpack1/5 -> BInvOnFRIn/1
  SPI Controller Transfer2/1 -> MATLAB Function2/1(RxBytes)
  MATLAB Function2/1(Message) -> CAN Unpack1/1
  SPI Controller Transfer8/1 -> MATLAB Function8/1(RxBytes)
  CAN Unpack1/8 -> BInvWarnFR/1
  CAN Unpack6/1 -> MMotorMeasuredFR/1
  CAN Unpack1/12 -> nMotorFR/1
  CAN Unpack1/4 -> BInvErrorFR/1
  CAN Unpack1/7 -> BInvSysReadyFR/1
  CAN Unpack1/9 -> BQuitInvOnFR/1
  Read RX Buffer start at RXB0SIDH2/1 -> SPI Controller Transfer2/1
  SPI Controller Transfer7/1 -> MATLAB Function7/1(RxBytes)
  Read RX Buffer start at RXB0SIDH8/1 -> SPI Controller Transfer8/1
  MATLAB Function6/1(Message) -> CAN Unpack6/1
  Read RX Buffer start at RXB0SIDH7/1 -> SPI Controller Transfer7/1
  CAN Unpack6/2 -> NInvDCTFR/1
  SPI Controller Transfer6/1 -> MATLAB Function6/1(RxBytes)
  MATLAB Function7/1(Message) -> CAN Unpack7/1
  Read RX Buffer start at RXB0SIDH6/1 -> SPI Controller Transfer6/1
  CAN Unpack7/4 -> VDCInvFR/1
  CAN Unpack8/4 -> TInvFR/1

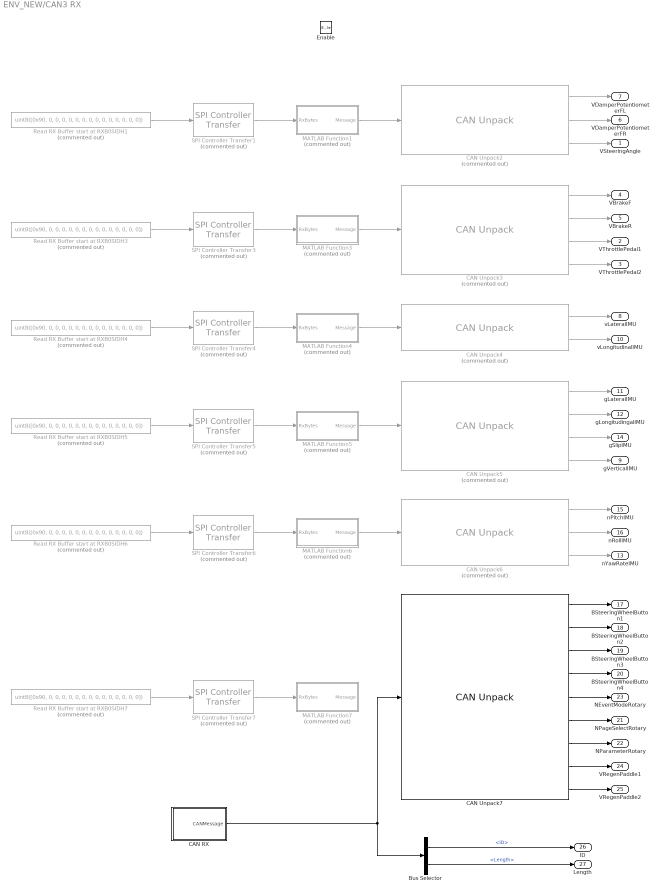
== system ENV_NEW/CAN3 RX ==
  Enable : EnablePort
  Bus Selector : BusSelector  OutputSignals=ID,Length
  CAN RX : Subsystem  mask{SPIModuleSelect=SPI1, Port_Select=GPIOA, Pin=1, PortName=GPIOA, PinNumber=2}
      mask prompts: SPIModuleSelect "SPI Module"; Port_Select "CS Port"; Pin "CS Pin"; PortName "INT Port"; PinNumber "INT Pin"
      mask TypeOptions SPIModuleSelect:
      | Enabled
      | Subsystem/SPI Controller Transfer7/SPIModuleSelect
      mask TypeOptions Port_Select:
      | Enabled
      | Subsystem/SPI Controller Transfer7/Port_Select
      mask TypeOptions Pin:
      | Enabled
      | Subsystem/SPI Controller Transfer7/Pin
      mask TypeOptions PortName: Digital Port Read5/PortName
      mask TypeOptions PinNumber: Digital Port Read5/PinNumber
      mask DialogControl DescTextVar Prompt: Read RX buffer when the INT pin is pulled low. Outputs a CANMessage type to be fed into a CAN unpack
      mask Display:
      | %port_label('output', 1, 'CANMessage');
      | 
      | text(0.05, 0.5, '' + string(get_param(gcb,'SPIModuleSelect')), HorizontalAlignment = 'left');
      | text(0.05, 0.85, 'CS ' + string(get_param(gcb,'Port_Select')) + ' Pin ' + string(get_param(gcb,'Pin')), HorizontalAlignment = 'left');
      | 
      | 
      | text(0.05, 0.15, 'INT ' + string(get_param(gcb,'PortName')) + ' Pin ' + string(get_param(gcb,'PinNumber')), HorizontalAlignment = 'left');
      | %text(0.05, 0.15, 'INT Pin ' + string(get_param(gcb,'PinNumber')), HorizontalAlignment = 'left');
      | 
      | 
      | % OBR logo
      | pos = get_param(gcb, 'Position');
      | blockAspect = (pos(3)-pos(1)) / (pos(4)-pos(2));
      | 
      | % fit(img, m, cx, cy): m = fraction of block the image occupies,
      | % (cx,cy) = center point in normalized 0-1 coords
      | fit = @(img,m,cx,cy) [ ...
      |     cx - m*min(1,(size(img,2)/size(img,1))/blockAspect)/2, ...
      |     cy - m*min(1,blockAspect/(size(img,2)/size(img,1)))/2, ...
      |     m*min(1,(size(img,2)/size(img,1))/blockAspect), ...
      |     m*min(1,blockAspect/(size(img,2)/size(img,1))) ];
      | 
      | ud = get_param(gcb, 'UserData');
      | 
      | image(ud.mcplogo, fit(ud.mcplogo, 0.3, 0.85, 0.5));
      | image(ud.obrlogo, fit(ud.obrlogo, 0.5, 0.5, 0.5));
  CAN Unpack2 : canmsglib/CAN Unpack  Commented=on  CANdbFile=C:\Users\oxbro\Documents\STM32CustomProjects\VCUSTM32\OBR26_Controls_30-7-26\CAN\CAN3\CAN3_03.08.26.dbc  MsgList=(none)  MsgName=DDU7_SteerDamper  MsgIDType=Standard (11-bit identifier)  MsgIdentifier=257  MsgLength=8  SignalInfo={'VDamperPotentiometerFL','16','13','LE','unsigned','Standard','0','1','0','0','8191';'VDamperPotentiometerFR','29','13','LE','unsigned','Standard','0','1','0','0','8191';'VSteeringAngle','0','13','LE','unsigned','Standard','0','1','0','0','8191'}  IDPort=off  TimestampPort=off  ErrorPort=off  RemotePort=off  LengthPort=off  StatusPort=off  ApplyMinMax=off
      settings: LibrarySourceBlock=stmutilitieslib/CAN Unpack  DataFormat=CANdb specified signals
  CAN Unpack3 : canmsglib/CAN Unpack  Commented=on  CANdbFile=C:\Users\oxbro\Documents\STM32CustomProjects\VCUSTM32\OBR26_Controls_30-7-26\CAN\CAN3\CAN3_03.08.26.dbc  MsgList=(none)  MsgName=DDU7_ThrBrake  MsgIDType=Standard (11-bit identifier)  MsgIdentifier=256  MsgLength=8  SignalInfo={'VBrakeF','0','16','LE','unsigned','Standard','0','1','0','0','3276.75';'VBrakeR','16','16','LE','unsigned','Standard','0','1','0','0','65535';'VThrottlePedal1','32','16','LE','unsigned','Standard','0','1','0','0','65535';'VThrottlePedal2','48','16','LE','unsigned','Standard','0','1','0','0','65535'}  IDPort=off  TimestampPort=off  ErrorPort=off  RemotePort=off  LengthPort=off  StatusPort=off  ApplyMinMax=off
      settings: LibrarySourceBlock=stmutilitieslib/CAN Unpack  DataFormat=CANdb specified signals
  CAN Unpack4 : canmsglib/CAN Unpack  Commented=on  CANdbFile=C:\Users\oxbro\Documents\STM32CustomProjects\VCUSTM32\OBR26_Controls_30-7-26\CAN\CAN3\CAN3_03.08.26.dbc  MsgList=(none)  MsgName=IMU_0x604  MsgIDType=Standard (11-bit identifier)  MsgIdentifier=1540  MsgLength=8  SignalInfo={'vLateralIMU','16','16','LE','signed','Standard','0','0.01','0','-327.68','327.67';'vLongitudinalIMU','0','16','LE','signed','Standard','0','0.01','0','-327.68','327.67'}  IDPort=off  TimestampPort=off  ErrorPort=off  RemotePort=off  LengthPort=off  StatusPort=off  ApplyMinMax=off
      settings: LibrarySourceBlock=stmutilitieslib/CAN Unpack  DataFormat=CANdb specified signals
  CAN Unpack5 : canmsglib/CAN Unpack  Commented=on  CANdbFile=C:\Users\oxbro\Documents\STM32CustomProjects\VCUSTM32\OBR26_Controls_30-7-26\CAN\CAN3\CAN3_03.08.26.dbc  MsgList=(none)  MsgName=IMU_0x606  MsgIDType=Standard (11-bit identifier)  MsgIdentifier=1542  MsgLength=8  SignalInfo={'gLateralIMU','16','16','LE','signed','Standard','0','0.01','0','-327.68','327.67';'gLongitudinalIMU','0','16','LE','signed','Standard','0','0.01','0','-327.68','327.67';'gSlipIMU','48','16','LE','signed','Standard','0','0.01','0','-327.68','327.67';'gVerticalIMU','32','16','LE','signed','Standard','0','0.01','0','-327.68','327.67'}  IDPort=off  TimestampPort=off  ErrorPort=off  RemotePort=off  LengthPort=off  StatusPort=off  ApplyMinMax=off
      settings: LibrarySourceBlock=stmutilitieslib/CAN Unpack  DataFormat=CANdb specified signals
  CAN Unpack6 : canmsglib/CAN Unpack  Commented=on  CANdbFile=C:\Users\oxbro\Documents\STM32CustomProjects\VCUSTM32\OBR26_Controls_30-7-26\CAN\CAN3\CAN3_03.08.26.dbc  MsgList=(none)  MsgName=IMU_0x609  MsgIDType=Standard (11-bit identifier)  MsgIdentifier=1545  MsgLength=8  SignalInfo={'nPitchIMU','16','16','LE','signed','Standard','0','0.01','0','-327.68','327.67';'nRollIMU','0','16','LE','signed','Standard','0','0.01','0','-327.68','327.67';'nYawRateIMU','32','16','LE','signed','Standard','0','0.01','0','-327.68','327.67'}  IDPort=off  TimestampPort=off  ErrorPort=off  RemotePort=off  LengthPort=off  StatusPort=off  ApplyMinMax=off
      settings: LibrarySourceBlock=stmutilitieslib/CAN Unpack  DataFormat=CANdb specified signals
  CAN Unpack7 : canmsglib/CAN Unpack  CANdbFile=C:\Users\oxbro\Documents\STM32CustomProjects\VCUSTM32\OBR26_Controls_30-7-26\CAN\CAN3\CAN3_03.08.26.dbc  MsgList=STW_0x1FB  MsgName=STW_0x1FB  MsgIDType=Standard (11-bit identifier)  MsgIdentifier=507  MsgLength=6  SignalInfo={'BSteeringWheelButton1','0','1','LE','unsigned','Standard','0','1','0','0','1';'BSteeringWheelButton2','1','1','LE','unsigned','Standard','0','1','0','0','1';'BSteeringWheelButton3','2','1','LE','unsigned','Standard','0','1','0','0','1';'BSteeringWheelButton4','3','1','LE','unsigned','Standard','0','1','0','0','1';'NEventModeRotary','20','8','LE','unsigned','Standard','0','1','1','1','16';'NPageSelectRotary','4','8','LE','unsigned','Standard','0','1','1','1','16';'NParameterRotary','12','8','LE','unsigned','Standard','0','1','1','1','16';'VRegenPaddle1','28','8','LE','unsigned','Standard','0','0.0129','0','0','3.2895';'VRegenPaddle2','36','8','LE','unsigned','Standard','0','0.0129','0','0','3.2895'}  IDPort=off  TimestampPort=off  ErrorPort=off  RemotePort=off  LengthPort=off  StatusPort=off  ApplyMinMax=off
      settings: LibrarySourceBlock=stmutilitieslib/CAN Unpack  DataFormat=CANdb specified signals
  MATLAB Function1 : MATLAB Function  Commented=on  TreatAsAtomicUnit=on
  MATLAB Function3 : MATLAB Function  Commented=on  TreatAsAtomicUnit=on
  MATLAB Function4 : MATLAB Function  Commented=on  TreatAsAtomicUnit=on
  MATLAB Function5 : MATLAB Function  Commented=on  TreatAsAtomicUnit=on
  MATLAB Function6 : MATLAB Function  Commented=on  TreatAsAtomicUnit=on
  MATLAB Function7 : MATLAB Function  Commented=on  TreatAsAtomicUnit=on
  Read RX Buffer start at RXB0SIDH{1,3..7} (6 alike) : Constant  Commented=on  Value=uint8([0x90, 0, 0, 0, 0, 0, 0, 0, 0, 0, 0, 0, 0, 0, 0])
  SPI Controller Transfer{1,3..7} (6 alike) : stm32blockslib/SPI Controller Transfer  Priority=1  Commented=on  SPIModuleSelect=SPI1  ClockPolarity=Low  ClockPhase=1 Edge  SPIModule=uint32(0)  Mode=Master  BusSpeed=uint32(1000000)  FirstBitToTransfer=Most significant bit (MSB)  ClockMode=0  BlockFunction=Transfer  EnableRegisterAddress=off  RegisterAddress=0  OutputDataType=uint8  OutputDataLength=1  OutputStatus=off  BlockingMode=on  Timeout=0.01  DataBits=8  UseCustomSSPin=Explicit GPIO calls  ActiveLowSSPin=Active low  Port_Select=GPIOA  Pin=1
      settings: LibrarySourceBlock=stm32h7xxblockslib/SPI Controller Transfer
  VSteeringAngle : Outport  OutDataTypeStr=double
  VThrottlePedal1 : Outport  Port=2  OutDataTypeStr=double
  VThrottlePedal2 : Outport  Port=3  OutDataTypeStr=double
  VBrakeF : Outport  Port=4  OutDataTypeStr=double
  VBrakeR : Outport  Port=5  OutDataTypeStr=double
  VDamperPotentiometerFR : Outport  Port=6  OutDataTypeStr=double
  VDamperPotentiometerFL : Outport  Port=7  OutDataTypeStr=double
  vLateralIMU : Outport  Port=8  OutDataTypeStr=double
  gVerticalIMU : Outport  Port=9  OutDataTypeStr=double
  vLongitudinalIMU : Outport  Port=10  OutDataTypeStr=double
  gLateralIMU : Outport  Port=11  OutDataTypeStr=double
  gLongitudingalIMU : Outport  Port=12  OutDataTypeStr=double
  nYawRateIMU : Outport  Port=13  OutDataTypeStr=double
  gSlipIMU : Outport  Port=14  OutDataTypeStr=double
  nPitchIMU : Outport  Port=15  OutDataTypeStr=double
  nRollIMU : Outport  Port=16  OutDataTypeStr=double
  BSteeringWheelButton1 : Outport  Port=17  OutDataTypeStr=boolean
  BSteeringWheelButton2 : Outport  Port=18  OutDataTypeStr=boolean
  BSteeringWheelButton3 : Outport  Port=19  OutDataTypeStr=boolean
  BSteeringWheelButton4 : Outport  Port=20  OutDataTypeStr=boolean
  NPageSelectRotary : Outport  Port=21  OutDataTypeStr=double
  NParameterRotary : Outport  Port=22  OutDataTypeStr=double
  NEventModeRotary : Outport  Port=23  OutDataTypeStr=double
  VRegenPaddle1 : Outport  Port=24  OutDataTypeStr=double
  VRegenPaddle2 : Outport  Port=25  OutDataTypeStr=double
  ID : Outport  Port=26
  Length : Outport  Port=27
  wires:
  Bus Selector/1 -> ID/1  "<ID>"
  Bus Selector/2 -> Length/1  "<Length>"
  CAN Unpack4/1 -> vLateralIMU/1
  CAN Unpack7/5 -> NEventModeRotary/1
  CAN Unpack7/3 -> BSteeringWheelButton3/1
  CAN Unpack2/1 -> VDamperPotentiometerFL/1
  CAN Unpack2/2 -> VDamperPotentiometerFR/1
  CAN Unpack5/4 -> gVerticalIMU/1
  CAN Unpack3/3 -> VThrottlePedal1/1
  CAN Unpack2/3 -> VSteeringAngle/1
  CAN Unpack6/2 -> nRollIMU/1
  CAN Unpack7/6 -> NPageSelectRotary/1
  CAN Unpack7/1 -> BSteeringWheelButton1/1
  CAN Unpack6/3 -> nYawRateIMU/1
  CAN Unpack3/1 -> VBrakeF/1
  CAN Unpack5/2 -> gLongitudingalIMU/1
  CAN Unpack7/9 -> VRegenPaddle2/1
  CAN Unpack7/7 -> NParameterRotary/1
  CAN Unpack7/2 -> BSteeringWheelButton2/1
  CAN Unpack3/4 -> VThrottlePedal2/1
  CAN Unpack3/2 -> VBrakeR/1
  CAN Unpack7/8 -> VRegenPaddle1/1
  CAN Unpack6/1 -> nPitchIMU/1
  CAN Unpack5/3 -> gSlipIMU/1
  CAN Unpack7/4 -> BSteeringWheelButton4/1
  CAN Unpack4/2 -> vLongitudinalIMU/1
  CAN Unpack5/1 -> gLateralIMU/1
  Read RX Buffer start at RXB0SIDH1/1 -> SPI Controller Transfer1/1
  SPI Controller Transfer1/1 -> MATLAB Function1/1(RxBytes)
  MATLAB Function1/1(Message) -> CAN Unpack2/1
  MATLAB Function3/1(Message) -> CAN Unpack3/1
  Read RX Buffer start at RXB0SIDH3/1 -> SPI Controller Transfer3/1
  SPI Controller Transfer3/1 -> MATLAB Function3/1(RxBytes)
  MATLAB Function4/1(Message) -> CAN Unpack4/1
  Read RX Buffer start at RXB0SIDH4/1 -> SPI Controller Transfer4/1
  SPI Controller Transfer4/1 -> MATLAB Function4/1(RxBytes)
  Read RX Buffer start at RXB0SIDH5/1 -> SPI Controller Transfer5/1
  SPI Controller Transfer5/1 -> MATLAB Function5/1(RxBytes)
  MATLAB Function5/1(Message) -> CAN Unpack5/1
  Read RX Buffer start at RXB0SIDH6/1 -> SPI Controller Transfer6/1
  SPI Controller Transfer6/1 -> MATLAB Function6/1(RxBytes)
  MATLAB Function6/1(Message) -> CAN Unpack6/1
  Read RX Buffer start at RXB0SIDH7/1 -> SPI Controller Transfer7/1
  SPI Controller Transfer7/1 -> MATLAB Function7/1(RxBytes)
  CAN RX/1(CANMessage) -> CAN Unpack7/1, Bus Selector/1
